simulink model "APP_DD11"  (R2016b)
settings: configuration reference "CodeGenConfigSet" (kept outside this file)
values from neighbouring files (symbols this model uses):
  APP_tiSRCHighDefDeb_C = Calibration.Parameter    [init_APP_DD1.m]
  APP_tiSRCHighOKDeb_C = Calibration.Parameter    [init_APP_DD1.m]
  APP_tiSRCLowDefDeb_C = Calibration.Parameter    [init_APP_DD1.m]
  APP_tiSRCLowOKDeb_C = Calibration.Parameter    [init_APP_DD1.m]
  APP_uRaw1Def_C = Calibration.Parameter    [init_APP_DD1.m]
  APP_uRaw1SRCHigh_C = Calibration.Parameter    [init_APP_DD1.m]
  APP_uRaw1SRCLow_C = Calibration.Parameter    [init_APP_DD1.m]
undefined symbols (not defined in the file or in its folder): APP_DD1_DT
libraries: CXLib x6
settings Model: Creator=lenovo  LastModifiedBy=lenovo
settings ConfigSetRef: SourceLocation=Base Workspace

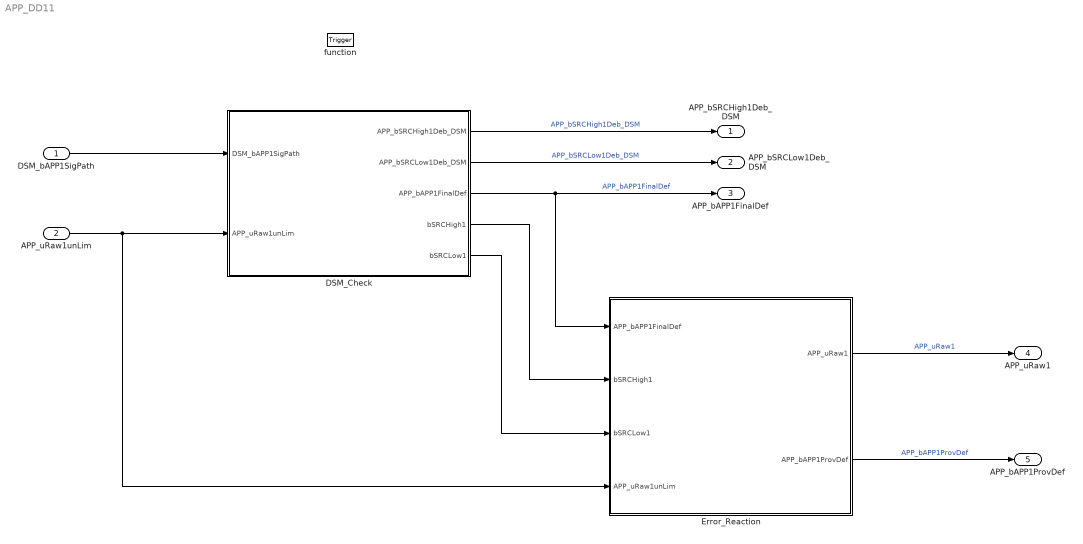
== system APP_DD11 ==
  DSM_bAPP1SigPath : Inport  Description=status of FId_APP1SigPath  OutMin=0  OutMax=1  OutDataTypeStr=boolean
  APP_uRaw1unLim : Inport  Tag=mv  Description=Acceleration pedal sensor 1 unlimited raw value  Port=2  OutMin=0  OutMax=5000  OutDataTypeStr=Ad_mv
  function : TriggerPort  TriggerType=function-call  VariantControl=Variant
  DSM_Check : Subsystem
  "Error_Reaction " : Subsystem
  APP_bSRCHigh1Deb_DSM : Outport  Description=Status debounced SRC-High error Sensor 1  OutMin=0  OutMax=1  OutDataTypeStr=boolean
  APP_bSRCLow1Deb_DSM : Outport  Description=Status debounced SRC-Low error Sensor 1  Port=2  OutMin=0  OutMax=1  OutDataTypeStr=boolean
  APP_bAPP1FinalDef : Outport  Description=Status Sensor 1 of the acceleration pedal finally defect  Port=3  OutMin=0  OutMax=1  OutDataTypeStr=boolean
  APP_uRaw1 : Outport  Tag=mv  Description=Acceleration Pedal Position D  Port=4  OutMin=0  OutMax=5000  OutDataTypeStr=Ad_mv
  APP_bAPP1ProvDef : Outport  Description=Status Sensor 1 of the acceleration pedal temporary defect  Port=5  OutMin=0  OutMax=1  OutDataTypeStr=boolean
  wires:
  DSM_Check/3(APP_bAPP1FinalDef) -> "Error_Reaction "/1(APP_bAPP1FinalDef), APP_bAPP1FinalDef/1  "APP_bAPP1FinalDef"
  DSM_bAPP1SigPath/1 -> DSM_Check/1(DSM_bAPP1SigPath)
  APP_uRaw1unLim/1 -> "Error_Reaction "/4(APP_uRaw1unLim), DSM_Check/2(APP_uRaw1unLim)
  DSM_Check/1(APP_bSRCHigh1Deb_DSM) -> APP_bSRCHigh1Deb_DSM/1  "APP_bSRCHigh1Deb_DSM"
  DSM_Check/2(APP_bSRCLow1Deb_DSM) -> APP_bSRCLow1Deb_DSM/1  "APP_bSRCLow1Deb_DSM"
  DSM_Check/4(bSRCHigh1) -> "Error_Reaction "/2(bSRCHigh1)
  DSM_Check/5(bSRCLow1) -> "Error_Reaction "/3(bSRCLow1)
  "Error_Reaction "/1(APP_uRaw1) -> APP_uRaw1/1  "APP_uRaw1"
  "Error_Reaction "/2(APP_bAPP1ProvDef) -> APP_bAPP1ProvDef/1  "APP_bAPP1ProvDef"

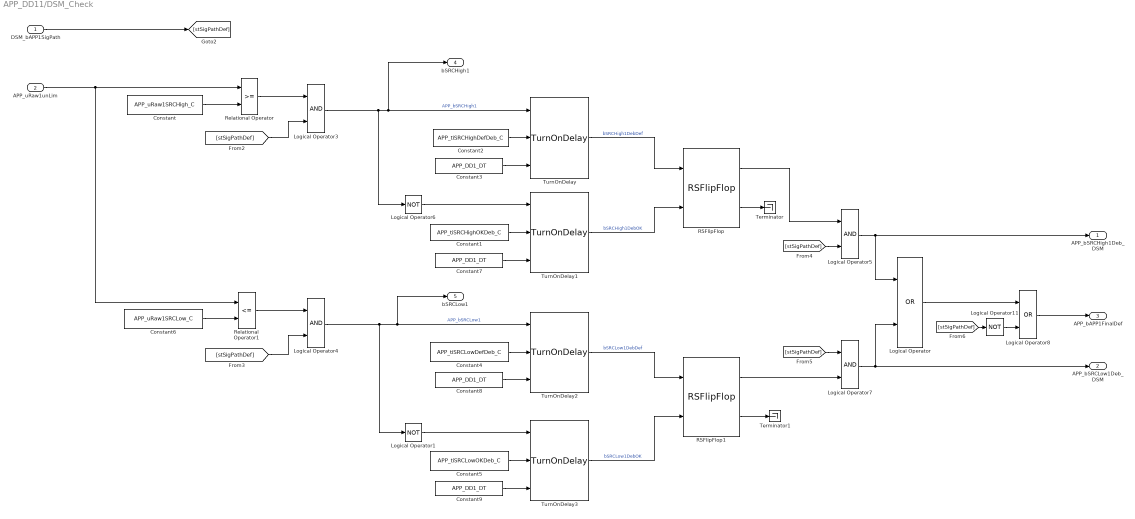
== system APP_DD11/DSM_Check ==
  DSM_bAPP1SigPath : Inport  Tag=-  Description=status of FId_APP1SigPath  OutMin=0  OutMax=1  OutDataTypeStr=boolean
  APP_uRaw1unLim : Inport  Tag=mv  Description=Acceleration pedal sensor 1 unlimited raw value  Port=2  OutMin=0  OutMax=5000  OutDataTypeStr=Ad_mv
  Constant : Constant  Value=APP_uRaw1SRCHigh_C
  Constant1 : Constant  Value=APP_tiSRCHighOKDeb_C
  Constant2 : Constant  Value=APP_tiSRCHighDefDeb_C
  Constant{3,7..9} (4 alike) : Constant  Value=APP_DD1_DT  OutDataTypeStr=Inherit: Inherit via back propagation
  Constant4 : Constant  Value=APP_tiSRCLowDefDeb_C
  Constant5 : Constant  Value=APP_tiSRCLowOKDeb_C
  Constant6 : Constant  Value=APP_uRaw1SRCLow_C
  Logical Operator : Logic  Operator=OR  AllPortsSameDT=off  OutDataTypeStr=boolean
  Logical Operator1 : Logic  Operator=NOT  AllPortsSameDT=off  OutDataTypeStr=boolean
  Logical Operator11 : Logic  Operator=NOT  AllPortsSameDT=off  OutDataTypeStr=boolean
  Logical Operator{3..5,7} (4 alike) : Logic  AllPortsSameDT=off  OutDataTypeStr=boolean
  Logical Operator6 : Logic  Operator=NOT  AllPortsSameDT=off  OutDataTypeStr=boolean
  Logical Operator8 : Logic  Operator=OR  AllPortsSameDT=off  OutDataTypeStr=boolean
  RSFlipFlop : CXLib/RSFlipFlop
  RSFlipFlop1 : CXLib/RSFlipFlop
  Relational Operator : RelationalOperator  OutDataTypeStr=boolean  RndMeth=Nearest  InputSameDT=on
  Relational Operator1 : RelationalOperator  Operator=<=  OutDataTypeStr=boolean  RndMeth=Nearest  InputSameDT=on
  Terminator : Terminator
  Terminator1 : Terminator
  TurnOnDelay{,1..3} (4 alike) : CXLib/TurnOnDelay
  APP_bSRCHigh1Deb_DSM : Outport  Tag=-  Description=Status debounced SRC-High error Sensor 1  OutMin=0  OutMax=1  OutDataTypeStr=boolean
  APP_bSRCLow1Deb_DSM : Outport  Tag=-  Description=Status debounced SRC-Low error Sensor 1  Port=2  OutMin=0  OutMax=1  OutDataTypeStr=boolean
  APP_bAPP1FinalDef : Outport  Tag=-  Description=Status Sensor 1 of the acceleration pedal finally defect  Port=3  OutMin=0  OutMax=1  OutDataTypeStr=boolean
  bSRCHigh1 : Outport  Port=4
  bSRCLow1 : Outport  Port=5
  wires:
  RSFlipFlop1/1 -> Logical Operator7/2
  RSFlipFlop/1 -> Logical Operator5/1
  Logical Operator1/1 -> TurnOnDelay3/1
  Logical Operator6/1 -> TurnOnDelay1/1
  Logical Operator11/1 -> Logical Operator8/2
  Logical Operator8/1 -> APP_bAPP1FinalDef/1
  [stSigPathDef] -> Logical Operator11/1
  Logical Operator/1 -> Logical Operator8/1
  [stSigPathDef] -> Logical Operator7/1
  [stSigPathDef] -> Logical Operator5/2
  [stSigPathDef] -> Logical Operator4/2
  Relational Operator1/1 -> Logical Operator4/1
  [stSigPathDef] -> Logical Operator3/2
  Relational Operator/1 -> Logical Operator3/1
  DSM_bAPP1SigPath/1 -> [stSigPathDef]
  Logical Operator7/1 -> APP_bSRCLow1Deb_DSM/1, Logical Operator/2
  Logical Operator5/1 -> APP_bSRCHigh1Deb_DSM/1, Logical Operator/1
  Logical Operator4/1 -> TurnOnDelay2/1, bSRCLow1/1, Logical Operator1/1  "APP_bSRCLow1"
  Constant6/1 -> Relational Operator1/2
  Logical Operator3/1 -> bSRCHigh1/1, TurnOnDelay/1, Logical Operator6/1  "APP_bSRCHigh1"
  Constant/1 -> Relational Operator/2
  APP_uRaw1unLim/1 -> Relational Operator/1, Relational Operator1/1
  Constant9/1 -> TurnOnDelay3/3
  Constant8/1 -> TurnOnDelay2/3
  Constant7/1 -> TurnOnDelay1/3
  Constant3/1 -> TurnOnDelay/3
  RSFlipFlop1/2 -> Terminator1/1
  RSFlipFlop/2 -> Terminator/1
  Constant5/1 -> TurnOnDelay3/2
  TurnOnDelay3/1 -> RSFlipFlop1/2  "bSRCLow1DebOK"
  TurnOnDelay2/1 -> RSFlipFlop1/1  "bSRCLow1DebDef"
  TurnOnDelay/1 -> RSFlipFlop/1  "bSRCHigh1DebDef"
  Constant2/1 -> TurnOnDelay/2
  Constant1/1 -> TurnOnDelay1/2
  Constant4/1 -> TurnOnDelay2/2
  TurnOnDelay1/1 -> RSFlipFlop/2  "bSRCHigh1DebOK"

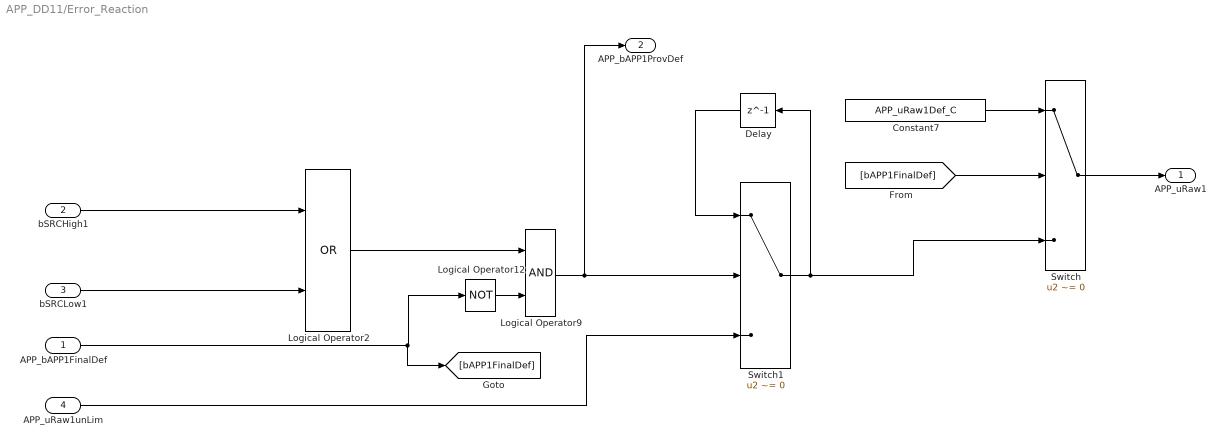
== system APP_DD11/Error_Reaction  ==
  APP_bAPP1FinalDef : Inport
  bSRCHigh1 : Inport  Port=2
  bSRCLow1 : Inport  Port=3
  APP_uRaw1unLim : Inport  Port=4
  Constant7 : Constant  Value=APP_uRaw1Def_C
  Delay : Delay  DelayLength=1  InitialCondition=0
  Logical Operator12 : Logic  Operator=NOT  AllPortsSameDT=off  OutDataTypeStr=boolean
  Logical Operator2 : Logic  Operator=OR  AllPortsSameDT=off  OutDataTypeStr=boolean
  Logical Operator9 : Logic  AllPortsSameDT=off  OutDataTypeStr=boolean
  Switch : Switch  Criteria=u2 ~= 0
  Switch1 : Switch  Criteria=u2 ~= 0
  APP_uRaw1 : Outport  Tag=mv  Description=Acceleration Pedal Position D  OutMin=0  OutMax=5000  OutDataTypeStr=Ad_mv
  APP_bAPP1ProvDef : Outport  Tag=-  Description=Status Sensor 1 of the acceleration pedal temporary defect  Port=2  OutMin=0  OutMax=1  OutDataTypeStr=boolean
  wires:
  Switch/1 -> APP_uRaw1/1
  Delay/1 -> Switch1/1
  Switch1/1 -> Delay/1, Switch/3
  Constant7/1 -> Switch/1
  Logical Operator12/1 -> Logical Operator9/2
  Logical Operator9/1 -> APP_bAPP1ProvDef/1, Switch1/2
  Logical Operator2/1 -> Logical Operator9/1
  bSRCLow1/1 -> Logical Operator2/2
  bSRCHigh1/1 -> Logical Operator2/1
  [bAPP1FinalDef] -> Switch/2
  APP_uRaw1unLim/1 -> Switch1/3
  APP_bAPP1FinalDef/1 -> [bAPP1FinalDef], Logical Operator12/1
